simulink model "conical_tank_system_behaviour_control101_2023"  (R2023b)
settings: Solver=ode45  StartTime=0.0  StopTime=endtime  RelTol=1e-3  EnableMultiTasking=on
undefined symbols (not defined in the file): alpha, beta, blockagetime, C, Ctemp, disturbanceflow, disturbanceflowtime, hss, itantheta2, qchangetime, qss, qstep
settings Model: Creator=stelios  LastModifiedBy=Anthony Rossiter
settings DataIOCC: LimitDataPoints=on  SaveFormat=Array  SignalLoggingSaveFormat=ModelDataLogs  ReturnWorkspaceOutputs=off
settings OptimizationCC: BooleanDataType=off
settings DebuggingCC: SaveWithParameterizedLinksMsg=none  UnderspecifiedInitializationDetection=Classic  MergeDetectMultiDrivingBlocksExec=none  SignalResolutionControl=TryResolveAllWithWarning  InheritedTsInSrcMsg=none  MultiTaskDSMMsg=warning  MultiTaskCondExecSysMsg=none  UnconnectedInputMsg=warning  UnconnectedOutputMsg=warning  UnconnectedLineMsg=warning
settings HardwareCC: TargetUnknown=on
settings ModelReferenceCC: EnableRefExpFcnMdlSchedulingChecks=on  PropagateSignalLabelsOutOfModel=off
settings RTWCC: DLArmComputeVersion=19.05
settings GRTTargetCC: CombineOutputUpdateFcns=off  GRTInterface=on
settings ConfigComp: CovMetricSettings=dw

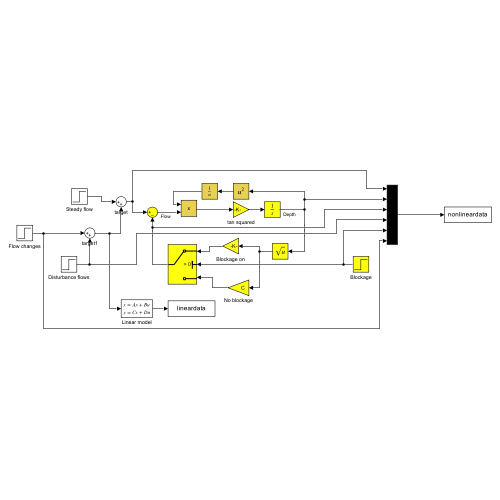
[thumbnail: Simulink's stored preview of the top-level diagram]
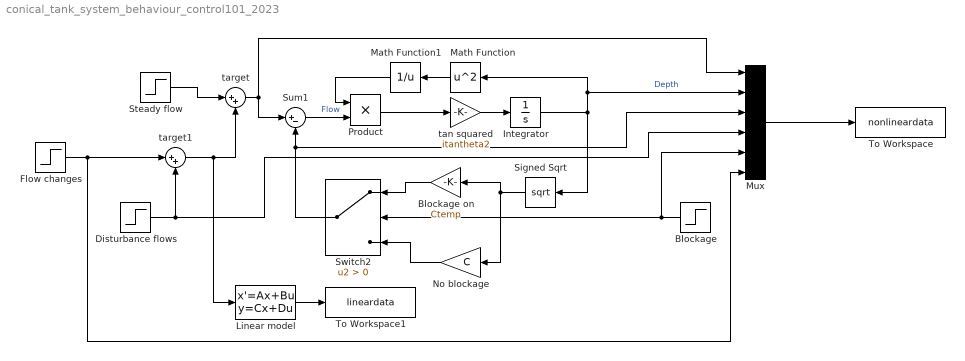
== system conical_tank_system_behaviour_control101_2023 ==
  Blockage : Step  Time=blockagetime
  Blockage on : Gain  Gain=Ctemp  SaturateOnIntegerOverflow=on
  Disturbance flows : Step  Time=disturbanceflowtime  After=disturbanceflow
  Flow changes : Step  Time=qchangetime  After=qstep
  Integrator : Integrator  InitialCondition=hss
  Linear model : StateSpace  A=beta  B=alpha  D=0  InitialCondition=0
  Math Function : Math  Operator=square
  Math Function1 : Math  Operator=reciprocal
  Mux : Mux  Inputs=6
  No blockage : Gain  Gain=C  SaturateOnIntegerOverflow=on
  Product : Product
  Signed Sqrt : Sqrt
  Steady flow : Step  Time=0  After=qss
  Sum1 : Sum  Inputs=|+-  SaturateOnIntegerOverflow=on
  Switch2 : Switch  Criteria=u2 > Threshold  SaturateOnIntegerOverflow=off  InputSameDT=off
  To Workspace : ToWorkspace  VariableName=nonlineardata  SaveFormat=Structure With Time  SampleTime=-1
  To Workspace1 : ToWorkspace  VariableName=lineardata  SaveFormat=Structure With Time  SampleTime=-1
  tan squared : Gain  Gain=itantheta2  SaturateOnIntegerOverflow=on
  target : Sum  Inputs=|++
  target1 : Sum  Inputs=|++
  wires:
  Mux/1 -> To Workspace/1
  Signed Sqrt/1 -> No blockage/1, Blockage on/1
  Integrator/1 -> Math Function/1, Mux/2, Signed Sqrt/1  "Depth"
  Blockage on/1 -> Switch2/1
  No blockage/1 -> Switch2/3
  Blockage/1 -> Mux/5, Switch2/2
  Steady flow/1 -> target/1
  Sum1/1 -> Product/2  "Flow"
  Product/1 -> tan squared/1
  tan squared/1 -> Integrator/1
  target/1 -> Mux/1, Sum1/1
  Math Function/1 -> Math Function1/1
  Math Function1/1 -> Product/1
  Switch2/1 -> Mux/3, Sum1/2
  Linear model/1 -> To Workspace1/1
  Flow changes/1 -> target1/1, Mux/6
  Disturbance flows/1 -> target1/2, Mux/4
  target1/1 -> Linear model/1, target/2
